simulink model "SecRwRtStFwdBkwdIsPosChk"  (R2024b)
settings: Solver=FixedStepDiscrete  StartTime=0.0  StopTime=10.0  FixedStep=0.01  RelTol=1e-3
undefined symbols (not defined in the file or in its folder): KeSMSuSecRwStFwdBkwdPosDelta_Val, KeSMSuSecRwStFwdBkwdPosTolr_Val
libraries: StIsPosChkLib x16, simulink x8
(part 2 of 2)

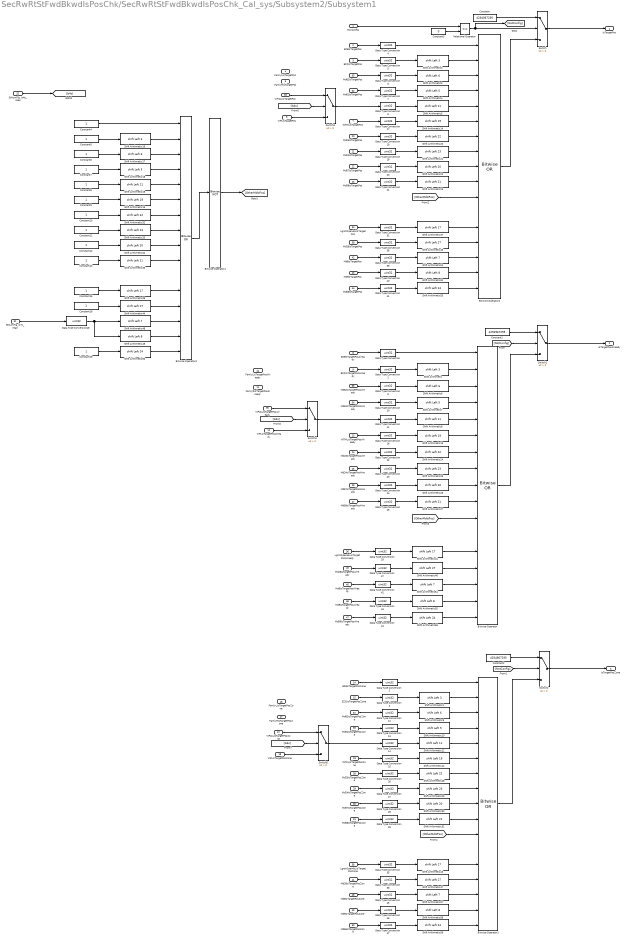
== system SecRwRtStFwdBkwdIsPosChk/SecRwRtStFwdBkwdIsPosChk_Cal_sys/Subsystem2/Subsystem1 ==
  MovConfig : Inport
  EZEIsTargetPos : Inport  Port=2
  EZQIsTargetPos : Inport  Port=3
  FamlyLIsTargetPos : Inport  Port=4
  FamlyRIsTargetPos : Inport  Port=5
  VIPLIsTargetPos : Inport  Port=6
  INTMLIsTargetPos : Inport  Port=7
  EZEIsTargetPosAlready : Inport  Port=8
  EZQIsTargetPosAlready : Inport  Port=9
  FamlyLIsTargetPosAlready : Inport  Port=10
  FamlyRIsTargetPosAlready : Inport  Port=11
  VIPLIsTargetPosAlready : Inport  Port=12
  INTMLIsTargetPosAlready : Inport  Port=13
  EZEIsTargetPosZone : Inport  Port=14
  EZQIsTargetPosZone : Inport  Port=15
  FamlyLIsTargetPosZone : Inport  Port=16
  FamlyRIsTargetPosZone : Inport  Port=17
  VIPLIsTargetPosZone : Inport  Port=18
  INTMLIsTargetPosZone : Inport  Port=19
  Md23IsTargetPos : Inport  Port=20
  Md24IsTargetPos : Inport  Port=21
  Md57IsTargetPos : Inport  Port=22
  Md58IsTargetPos : Inport  Port=23
  Md23IsTargetPosAlready : Inport  Port=24
  Md24IsTargetPosAlready : Inport  Port=25
  Md57IsTargetPosAlready : Inport  Port=26
  Md58IsTargetPosAlready : Inport  Port=27
  Md23IsTargetPosZone : Inport  Port=28
  Md24IsTargetPosZone : Inport  Port=29
  Md57IsTargetPosZone : Inport  Port=30
  Md58IsTargetPosZone : Inport  Port=31
  StNumFlg_Is4s_read : Inport  Port=32
  VIP4sLIsTargetPos : Inport  Port=33
  LgrstOpen4sLIsTargetPos : Inport  Port=34
  VIP4sLIsTargetPosAlready : Inport  Port=35
  LgrstOpen4sLIsTargetPosAlready : Inport  Port=36
  VIP4sLIsTargetPosZone : Inport  Port=37
  LgrstOpen4sLIsTargetPosZone : Inport  Port=38
  Md28IsTargetPos : Inport  Port=39
  Md28IsTargetPosAlready : Inport  Port=40
  Md28IsTargetPosZone : Inport  Port=41
  Md8IsTargetPos : Inport  Port=42
  Md9IsTargetPos : Inport  Port=43
  Md56IsTargetPos : Inport  Port=44
  Md8IsTargetPosAlready : Inport  Port=45
  Md9IsTargetPosAlready : Inport  Port=46
  Md56IsTargetPosAlready : Inport  Port=47
  Md8IsTargetPosZone : Inport  Port=48
  Md9IsTargetPosZone : Inport  Port=49
  Md56IsTargetPosZone : Inport  Port=50
  StNumFlg_Is7s_read : Inport  Port=51
  Md61IsTargetPos : Inport  Port=52
  Md62IsTargetPos : Inport  Port=53
  Md61IsTargetPosAlready : Inport  Port=54
  Md62IsTargetPosAlready : Inport  Port=55
  Md61IsTargetPosZone : Inport  Port=56
  Md62IsTargetPosZone : Inport  Port=57
  Bitwise Operator : simulink/Logic and Bit Operations/Bitwise Operator  logicop=OR  UseBitMask=off  NumInputPorts=17  BitMask=bin2dec('11011001')  BitMaskRealWorld=Stored Integer
  Bitwise Operator1 : simulink/Logic and Bit Operations/Bitwise Operator  logicop=OR  UseBitMask=off  NumInputPorts=17  BitMask=bin2dec('11011001')  BitMaskRealWorld=Stored Integer
  Bitwise Operator2 : simulink/Logic and Bit Operations/Bitwise Operator  logicop=OR  UseBitMask=off  NumInputPorts=17  BitMask=bin2dec('11011001')  BitMaskRealWorld=Stored Integer
  Bitwise Operator3 : simulink/Logic and Bit Operations/Bitwise Operator  logicop=OR  UseBitMask=off  NumInputPorts=16  BitMask=bin2dec('11011001')  BitMaskRealWorld=Stored Integer
  Bitwise Operator4 : simulink/Logic and Bit Operations/Bitwise Operator  logicop=NOT  UseBitMask=off  BitMask=bin2dec('11011001')  BitMaskRealWorld=Stored Integer
  Constant : Constant  Value=4294967295  OutDataTypeStr=uint32
  Constant1 : Constant  Value=4294967295  OutDataTypeStr=uint32
  Constant{4..13,15..16,19} (13 alike) : Constant  OutDataTypeStr=uint32
  Constant2 : Constant  Value=4294967295  OutDataTypeStr=uint32
  Constant3 : Constant  Value=0  OutDataTypeStr=uint8
  Data Type Conversion{,1..29,31,33,35..48} (46 alike) : DataTypeConversion  OutDataTypeStr=uint32  SaturateOnIntegerOverflow=off  RndMeth=Floor
  Relational Operator : RelationalOperator  Operator===  OutDataTypeStr=boolean  RndMeth=Simplest  InputSameDT=off
  Shift Arithmetic{,1..2,16} (4 alike) : ArithShift  BitShiftNumber=3  BitShiftDirection=Left
  Shift Arithmetic{4,7,10,18} (4 alike) : ArithShift  BitShiftNumber=5  BitShiftDirection=Left
  Shift Arithmetic{5,8,11,19} (4 alike) : ArithShift  BitShiftNumber=11  BitShiftDirection=Left
  Shift Arithmetic{12..15} (4 alike) : ArithShift  BitShiftNumber=19  BitShiftDirection=Left
  Shift Arithmetic{3,6,9,17} (4 alike) : ArithShift  BitShiftNumber=6  BitShiftDirection=Left
  Shift Arithmetic{20,24,28,32} (4 alike) : ArithShift  BitShiftNumber=22  BitShiftDirection=Left
  Shift Arithmetic{21,25,29,33} (4 alike) : ArithShift  BitShiftNumber=23  BitShiftDirection=Left
  Shift Arithmetic{22,26,30,34} (4 alike) : ArithShift  BitShiftNumber=20  BitShiftDirection=Left
  Shift Arithmetic{23,27,31,35} (4 alike) : ArithShift  BitShiftNumber=21  BitShiftDirection=Left
  Shift Arithmetic{37,39,41,43} (4 alike) : ArithShift  BitShiftNumber=17  BitShiftDirection=Left
  Shift Arithmetic{44..47} (4 alike) : ArithShift  BitShiftNumber=27  BitShiftDirection=Left
  Shift Arithmetic{48,51,54,57} (4 alike) : ArithShift  BitShiftNumber=7  BitShiftDirection=Left
  Shift Arithmetic{49,52,55,58} (4 alike) : ArithShift  BitShiftNumber=8  BitShiftDirection=Left
  Shift Arithmetic{50,53,56,59} (4 alike) : ArithShift  BitShiftNumber=24  BitShiftDirection=Left
  Switch{,1..5} (6 alike) : Switch  Criteria=u2 > Threshold  SaturateOnIntegerOverflow=off  InputSameDT=off
  IsTargetPos : Outport  VectorParamsAs1DForOutWhenUnconnected=off
      settings: EnsureOutportIsVirtual=on
  IsTargetPosAlready : Outport  Port=2  VectorParamsAs1DForOutWhenUnconnected=off
      settings: EnsureOutportIsVirtual=on
  IsTargetPosZone : Outport  Port=3  VectorParamsAs1DForOutWhenUnconnected=off
      settings: EnsureOutportIsVirtual=on
  wires:
  Constant3/1 -> Relational Operator/2
  Constant/1 -> Switch/1
  Relational Operator/1 -> [NotConfig], Switch/2
  MovConfig/1 -> Relational Operator/1
  Switch/1 -> IsTargetPos/1
  [NotConfig] -> Switch1/2
  Constant1/1 -> Switch1/1
  Switch1/1 -> IsTargetPosAlready/1
  Switch2/1 -> IsTargetPosZone/1
  Constant2/1 -> Switch2/1
  [NotConfig] -> Switch2/2
  Data Type Conversion1/1 -> Shift Arithmetic/1
  Data Type Conversion/1 -> Bitwise Operator/1
  Shift Arithmetic/1 -> Bitwise Operator/2
  Shift Arithmetic1/1 -> Bitwise Operator1/2
  Data Type Conversion2/1 -> Bitwise Operator1/1
  Data Type Conversion3/1 -> Shift Arithmetic1/1
  Bitwise Operator1/1 -> Switch2/3
  Bitwise Operator/1 -> Switch1/3
  Shift Arithmetic2/1 -> Bitwise Operator2/2
  Data Type Conversion4/1 -> Bitwise Operator2/1
  Data Type Conversion5/1 -> Shift Arithmetic2/1
  Bitwise Operator2/1 -> Switch/3
  EZEIsTargetPos/1 -> Data Type Conversion4/1
  EZQIsTargetPos/1 -> Data Type Conversion5/1
  EZQIsTargetPosZone/1 -> Data Type Conversion3/1
  EZEIsTargetPosZone/1 -> Data Type Conversion2/1
  EZQIsTargetPosAlready/1 -> Data Type Conversion1/1
  EZEIsTargetPosAlready/1 -> Data Type Conversion/1
  Shift Arithmetic3/1 -> Bitwise Operator2/3
  Shift Arithmetic4/1 -> Bitwise Operator2/4
  Shift Arithmetic5/1 -> Bitwise Operator2/5
  Data Type Conversion7/1 -> Shift Arithmetic4/1
  Data Type Conversion6/1 -> Shift Arithmetic3/1
  Data Type Conversion8/1 -> Shift Arithmetic5/1
  Data Type Conversion11/1 -> Shift Arithmetic8/1
  Data Type Conversion9/1 -> Shift Arithmetic6/1
  Data Type Conversion10/1 -> Shift Arithmetic7/1
  Shift Arithmetic8/1 -> Bitwise Operator/5
  Shift Arithmetic7/1 -> Bitwise Operator/4
  Shift Arithmetic6/1 -> Bitwise Operator/3
  Data Type Conversion14/1 -> Shift Arithmetic11/1
  Data Type Conversion13/1 -> Shift Arithmetic10/1
  Shift Arithmetic10/1 -> Bitwise Operator1/4
  Shift Arithmetic9/1 -> Bitwise Operator1/3
  Shift Arithmetic11/1 -> Bitwise Operator1/5
  Data Type Conversion12/1 -> Shift Arithmetic9/1
  Shift Arithmetic12/1 -> Bitwise Operator1/6
  Data Type Conversion15/1 -> Shift Arithmetic12/1
  INTMLIsTargetPosZone/1 -> Data Type Conversion15/1
  Shift Arithmetic13/1 -> Bitwise Operator/6
  Data Type Conversion16/1 -> Shift Arithmetic13/1
  INTMLIsTargetPosAlready/1 -> Data Type Conversion16/1
  Shift Arithmetic14/1 -> Bitwise Operator2/6
  Data Type Conversion17/1 -> Shift Arithmetic14/1
  INTMLIsTargetPos/1 -> Data Type Conversion17/1
  Shift Arithmetic15/1 -> Bitwise Operator3/6
  Shift Arithmetic18/1 -> Bitwise Operator3/4
  Shift Arithmetic17/1 -> Bitwise Operator3/3
  Bitwise Operator3/1 -> Bitwise Operator4/1
  Constant4/1 -> Bitwise Operator3/1
  Shift Arithmetic16/1 -> Bitwise Operator3/2
  Constant5/1 -> Shift Arithmetic16/1
  Constant6/1 -> Shift Arithmetic17/1
  Constant7/1 -> Shift Arithmetic18/1
  Constant8/1 -> Shift Arithmetic19/1
  Constant9/1 -> Shift Arithmetic15/1
  Bitwise Operator4/1 -> [OtherMdIsPos]
  [OtherMdIsPos] -> Bitwise Operator2/11
  Md23IsTargetPos/1 -> Data Type Conversion18/1
  Data Type Conversion18/1 -> Shift Arithmetic20/1
  Shift Arithmetic20/1 -> Bitwise Operator2/7
  Shift Arithmetic21/1 -> Bitwise Operator2/8
  Data Type Conversion19/1 -> Shift Arithmetic21/1
  Md24IsTargetPos/1 -> Data Type Conversion19/1
  Md57IsTargetPos/1 -> Data Type Conversion20/1
  Data Type Conversion20/1 -> Shift Arithmetic22/1
  Shift Arithmetic22/1 -> Bitwise Operator2/9
  Data Type Conversion21/1 -> Shift Arithmetic23/1
  Md58IsTargetPos/1 -> Data Type Conversion21/1
  Shift Arithmetic23/1 -> Bitwise Operator2/10
  [OtherMdIsPos] -> Bitwise Operator/11
  Md23IsTargetPosAlready/1 -> Data Type Conversion22/1
  Data Type Conversion22/1 -> Shift Arithmetic24/1
  Shift Arithmetic24/1 -> Bitwise Operator/7
  Shift Arithmetic25/1 -> Bitwise Operator/8
  Data Type Conversion23/1 -> Shift Arithmetic25/1
  Md24IsTargetPosAlready/1 -> Data Type Conversion23/1
  Md57IsTargetPosAlready/1 -> Data Type Conversion24/1
  Data Type Conversion24/1 -> Shift Arithmetic26/1
  Shift Arithmetic26/1 -> Bitwise Operator/9
  Shift Arithmetic27/1 -> Bitwise Operator/10
  Data Type Conversion25/1 -> Shift Arithmetic27/1
  Md58IsTargetPosAlready/1 -> Data Type Conversion25/1
  [OtherMdIsPos] -> Bitwise Operator1/11
  Md23IsTargetPosZone/1 -> Data Type Conversion26/1
  Data Type Conversion26/1 -> Shift Arithmetic28/1
  Shift Arithmetic28/1 -> Bitwise Operator1/7
  Shift Arithmetic29/1 -> Bitwise Operator1/8
  Data Type Conversion27/1 -> Shift Arithmetic29/1
  Md24IsTargetPosZone/1 -> Data Type Conversion27/1
  Md57IsTargetPosZone/1 -> Data Type Conversion28/1
  Data Type Conversion28/1 -> Shift Arithmetic30/1
  Shift Arithmetic30/1 -> Bitwise Operator1/9
  Shift Arithmetic31/1 -> Bitwise Operator1/10
  Data Type Conversion29/1 -> Shift Arithmetic31/1
  Md58IsTargetPosZone/1 -> Data Type Conversion29/1
  Constant10/1 -> Shift Arithmetic32/1
  Shift Arithmetic32/1 -> Bitwise Operator3/7
  Constant11/1 -> Shift Arithmetic33/1
  Shift Arithmetic33/1 -> Bitwise Operator3/8
  Shift Arithmetic34/1 -> Bitwise Operator3/9
  Constant12/1 -> Shift Arithmetic34/1
  Constant13/1 -> Shift Arithmetic35/1
  Shift Arithmetic35/1 -> Bitwise Operator3/10
  Shift Arithmetic19/1 -> Bitwise Operator3/5
  StNumFlg_Is4s_read/1 -> [Is4s]
  VIP4sLIsTargetPos/1 -> Switch3/1
  [Is4s] -> Switch3/2
  VIPLIsTargetPos/1 -> Switch3/3
  Switch3/1 -> Data Type Conversion8/1
  Data Type Conversion31/1 -> Shift Arithmetic37/1
  LgrstOpen4sLIsTargetPos/1 -> Data Type Conversion31/1
  Shift Arithmetic37/1 -> Bitwise Operator2/13
  Shift Arithmetic39/1 -> Bitwise Operator3/12
  Constant15/1 -> Shift Arithmetic39/1
  Switch4/1 -> Data Type Conversion11/1
  [Is4s] -> Switch4/2
  VIP4sLIsTargetPosAlready/1 -> Switch4/1
  VIPLIsTargetPosAlready/1 -> Switch4/3
  Shift Arithmetic41/1 -> Bitwise Operator/13
  LgrstOpen4sLIsTargetPosAlready/1 -> Data Type Conversion33/1
  Data Type Conversion33/1 -> Shift Arithmetic41/1
  Data Type Conversion35/1 -> Shift Arithmetic43/1
  LgrstOpen4sLIsTargetPosZone/1 -> Data Type Conversion35/1
  Shift Arithmetic43/1 -> Bitwise Operator1/13
  VIP4sLIsTargetPosZone/1 -> Switch5/1
  [Is4s] -> Switch5/2
  Switch5/1 -> Data Type Conversion14/1
  VIPLIsTargetPosZone/1 -> Switch5/3
  Constant16/1 -> Shift Arithmetic44/1
  Shift Arithmetic44/1 -> Bitwise Operator3/13
  Shift Arithmetic45/1 -> Bitwise Operator2/14
  Md28IsTargetPos/1 -> Data Type Conversion36/1
  Data Type Conversion36/1 -> Shift Arithmetic45/1
  Data Type Conversion37/1 -> Shift Arithmetic46/1
  Md28IsTargetPosAlready/1 -> Data Type Conversion37/1
  Shift Arithmetic46/1 -> Bitwise Operator/14
  Shift Arithmetic47/1 -> Bitwise Operator1/14
  Md28IsTargetPosZone/1 -> Data Type Conversion38/1
  Data Type Conversion38/1 -> Shift Arithmetic47/1
  Shift Arithmetic48/1 -> Bitwise Operator3/14
  Data Type Conversion48/1 -> Shift Arithmetic49/1, Shift Arithmetic48/1
  Shift Arithmetic49/1 -> Bitwise Operator3/15
  Shift Arithmetic50/1 -> Bitwise Operator3/16
  Constant19/1 -> Shift Arithmetic50/1
  Data Type Conversion39/1 -> Shift Arithmetic51/1
  Md8IsTargetPos/1 -> Data Type Conversion39/1
  Shift Arithmetic51/1 -> Bitwise Operator2/15
  Shift Arithmetic52/1 -> Bitwise Operator2/16
  Md9IsTargetPos/1 -> Data Type Conversion40/1
  Data Type Conversion40/1 -> Shift Arithmetic52/1
  Data Type Conversion41/1 -> Shift Arithmetic53/1
  Md56IsTargetPos/1 -> Data Type Conversion41/1
  Shift Arithmetic53/1 -> Bitwise Operator2/17
  Shift Arithmetic54/1 -> Bitwise Operator/15
  Md8IsTargetPosAlready/1 -> Data Type Conversion42/1
  Data Type Conversion42/1 -> Shift Arithmetic54/1
  Data Type Conversion43/1 -> Shift Arithmetic55/1
  Md9IsTargetPosAlready/1 -> Data Type Conversion43/1
  Shift Arithmetic55/1 -> Bitwise Operator/16
  Shift Arithmetic56/1 -> Bitwise Operator/17
  Md56IsTargetPosAlready/1 -> Data Type Conversion44/1
  Data Type Conversion44/1 -> Shift Arithmetic56/1
  Data Type Conversion45/1 -> Shift Arithmetic57/1
  Md8IsTargetPosZone/1 -> Data Type Conversion45/1
  Shift Arithmetic57/1 -> Bitwise Operator1/15
  Shift Arithmetic58/1 -> Bitwise Operator1/16
  Md9IsTargetPosZone/1 -> Data Type Conversion46/1
  Data Type Conversion46/1 -> Shift Arithmetic58/1
  Data Type Conversion47/1 -> Shift Arithmetic59/1
  Md56IsTargetPosZone/1 -> Data Type Conversion47/1
  Shift Arithmetic59/1 -> Bitwise Operator1/17
  StNumFlg_Is7s_read/1 -> Data Type Conversion48/1
  Md61IsTargetPos/1 -> Data Type Conversion7/1
  Md62IsTargetPos/1 -> Data Type Conversion6/1
  Md61IsTargetPosAlready/1 -> Data Type Conversion10/1
  Md62IsTargetPosAlready/1 -> Data Type Conversion9/1
  Md61IsTargetPosZone/1 -> Data Type Conversion13/1
  Md62IsTargetPosZone/1 -> Data Type Conversion12/1

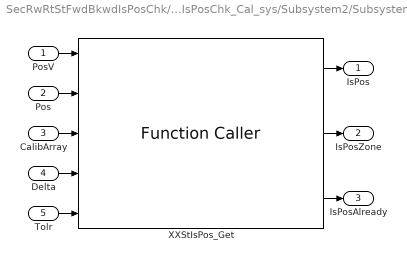
== system SecRwRtStFwdBkwdIsPosChk/SecRwRtStFwdBkwdIsPosChk_Cal_sys/Subsystem2/Subsystem10 ==
  PosV : Inport
  Pos : Inport  Port=2
  CalibArray : Inport  Port=3
  Delta : Inport  Port=4
  Tolr : Inport  Port=5
  XXStIsPos_Get : FunctionCaller  FunctionPrototype=[IsPos,IsPosZone,IsPosAlready] = XXStIsPos_Get(PosV,Pos,CalibArray,Delta,Tolr)  InputArgumentSpecifications=boolean(true), uint16(1), uint16([1;1;1]), uint16(1), uint16(1)  OutputArgumentSpecifications=boolean(true), boolean(true), boolean(true)
  IsPos : Outport  VectorParamsAs1DForOutWhenUnconnected=off
  IsPosZone : Outport  Port=2  VectorParamsAs1DForOutWhenUnconnected=off
  IsPosAlready : Outport  Port=3  VectorParamsAs1DForOutWhenUnconnected=off
  wires:
  Pos/1 -> XXStIsPos_Get/2
  PosV/1 -> XXStIsPos_Get/1
  XXStIsPos_Get/1 -> IsPos/1
  XXStIsPos_Get/2 -> IsPosZone/1
  CalibArray/1 -> XXStIsPos_Get/3
  XXStIsPos_Get/3 -> IsPosAlready/1
  Tolr/1 -> XXStIsPos_Get/5
  Delta/1 -> XXStIsPos_Get/4

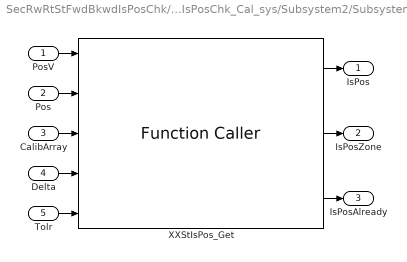
== system SecRwRtStFwdBkwdIsPosChk/SecRwRtStFwdBkwdIsPosChk_Cal_sys/Subsystem2/Subsystem11 ==
  PosV : Inport
  Pos : Inport  Port=2
  CalibArray : Inport  Port=3
  Delta : Inport  Port=4
  Tolr : Inport  Port=5
  XXStIsPos_Get : FunctionCaller  FunctionPrototype=[IsPos,IsPosZone,IsPosAlready] = XXStIsPos_Get(PosV,Pos,CalibArray,Delta,Tolr)  InputArgumentSpecifications=boolean(true), uint16(1), uint16([1;1;1]), uint16(1), uint16(1)  OutputArgumentSpecifications=boolean(true), boolean(true), boolean(true)
  IsPos : Outport  VectorParamsAs1DForOutWhenUnconnected=off
  IsPosZone : Outport  Port=2  VectorParamsAs1DForOutWhenUnconnected=off
  IsPosAlready : Outport  Port=3  VectorParamsAs1DForOutWhenUnconnected=off
  wires:
  Delta/1 -> XXStIsPos_Get/4
  Tolr/1 -> XXStIsPos_Get/5
  XXStIsPos_Get/3 -> IsPosAlready/1
  CalibArray/1 -> XXStIsPos_Get/3
  XXStIsPos_Get/2 -> IsPosZone/1
  XXStIsPos_Get/1 -> IsPos/1
  PosV/1 -> XXStIsPos_Get/1
  Pos/1 -> XXStIsPos_Get/2

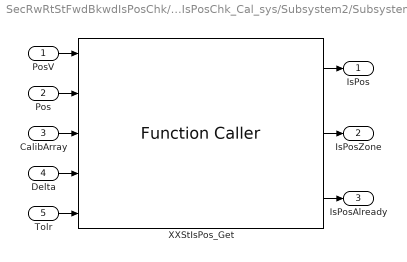
== system SecRwRtStFwdBkwdIsPosChk/SecRwRtStFwdBkwdIsPosChk_Cal_sys/Subsystem2/Subsystem12 ==
  PosV : Inport
  Pos : Inport  Port=2
  CalibArray : Inport  Port=3
  Delta : Inport  Port=4
  Tolr : Inport  Port=5
  XXStIsPos_Get : FunctionCaller  FunctionPrototype=[IsPos,IsPosZone,IsPosAlready] = XXStIsPos_Get(PosV,Pos,CalibArray,Delta,Tolr)  InputArgumentSpecifications=boolean(true), uint16(1), uint16([1;1;1]), uint16(1), uint16(1)  OutputArgumentSpecifications=boolean(true), boolean(true), boolean(true)
  IsPos : Outport  VectorParamsAs1DForOutWhenUnconnected=off
  IsPosZone : Outport  Port=2  VectorParamsAs1DForOutWhenUnconnected=off
  IsPosAlready : Outport  Port=3  VectorParamsAs1DForOutWhenUnconnected=off
  wires:
  Pos/1 -> XXStIsPos_Get/2
  PosV/1 -> XXStIsPos_Get/1
  XXStIsPos_Get/1 -> IsPos/1
  XXStIsPos_Get/2 -> IsPosZone/1
  CalibArray/1 -> XXStIsPos_Get/3
  XXStIsPos_Get/3 -> IsPosAlready/1
  Tolr/1 -> XXStIsPos_Get/5
  Delta/1 -> XXStIsPos_Get/4

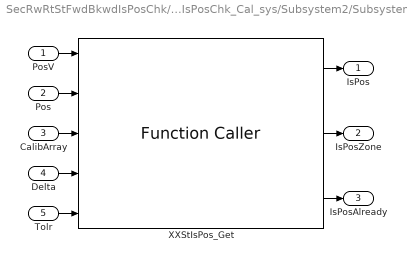
== system SecRwRtStFwdBkwdIsPosChk/SecRwRtStFwdBkwdIsPosChk_Cal_sys/Subsystem2/Subsystem13 ==
  PosV : Inport
  Pos : Inport  Port=2
  CalibArray : Inport  Port=3
  Delta : Inport  Port=4
  Tolr : Inport  Port=5
  XXStIsPos_Get : FunctionCaller  FunctionPrototype=[IsPos,IsPosZone,IsPosAlready] = XXStIsPos_Get(PosV,Pos,CalibArray,Delta,Tolr)  InputArgumentSpecifications=boolean(true), uint16(1), uint16([1;1;1]), uint16(1), uint16(1)  OutputArgumentSpecifications=boolean(true), boolean(true), boolean(true)
  IsPos : Outport  VectorParamsAs1DForOutWhenUnconnected=off
  IsPosZone : Outport  Port=2  VectorParamsAs1DForOutWhenUnconnected=off
  IsPosAlready : Outport  Port=3  VectorParamsAs1DForOutWhenUnconnected=off
  wires:
  Delta/1 -> XXStIsPos_Get/4
  Tolr/1 -> XXStIsPos_Get/5
  XXStIsPos_Get/3 -> IsPosAlready/1
  CalibArray/1 -> XXStIsPos_Get/3
  XXStIsPos_Get/2 -> IsPosZone/1
  XXStIsPos_Get/1 -> IsPos/1
  PosV/1 -> XXStIsPos_Get/1
  Pos/1 -> XXStIsPos_Get/2

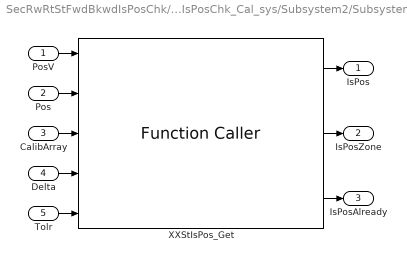
== system SecRwRtStFwdBkwdIsPosChk/SecRwRtStFwdBkwdIsPosChk_Cal_sys/Subsystem2/Subsystem14 ==
  PosV : Inport
  Pos : Inport  Port=2
  CalibArray : Inport  Port=3
  Delta : Inport  Port=4
  Tolr : Inport  Port=5
  XXStIsPos_Get : FunctionCaller  FunctionPrototype=[IsPos,IsPosZone,IsPosAlready] = XXStIsPos_Get(PosV,Pos,CalibArray,Delta,Tolr)  InputArgumentSpecifications=boolean(true), uint16(1), uint16([1;1;1]), uint16(1), uint16(1)  OutputArgumentSpecifications=boolean(true), boolean(true), boolean(true)
  IsPos : Outport  VectorParamsAs1DForOutWhenUnconnected=off
  IsPosZone : Outport  Port=2  VectorParamsAs1DForOutWhenUnconnected=off
  IsPosAlready : Outport  Port=3  VectorParamsAs1DForOutWhenUnconnected=off
  wires:
  Pos/1 -> XXStIsPos_Get/2
  PosV/1 -> XXStIsPos_Get/1
  XXStIsPos_Get/1 -> IsPos/1
  XXStIsPos_Get/2 -> IsPosZone/1
  CalibArray/1 -> XXStIsPos_Get/3
  XXStIsPos_Get/3 -> IsPosAlready/1
  Tolr/1 -> XXStIsPos_Get/5
  Delta/1 -> XXStIsPos_Get/4

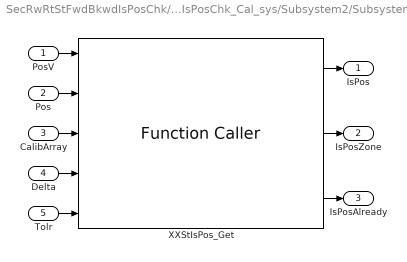
== system SecRwRtStFwdBkwdIsPosChk/SecRwRtStFwdBkwdIsPosChk_Cal_sys/Subsystem2/Subsystem15 ==
  PosV : Inport
  Pos : Inport  Port=2
  CalibArray : Inport  Port=3
  Delta : Inport  Port=4
  Tolr : Inport  Port=5
  XXStIsPos_Get : FunctionCaller  FunctionPrototype=[IsPos,IsPosZone,IsPosAlready] = XXStIsPos_Get(PosV,Pos,CalibArray,Delta,Tolr)  InputArgumentSpecifications=boolean(true), uint16(1), uint16([1;1;1]), uint16(1), uint16(1)  OutputArgumentSpecifications=boolean(true), boolean(true), boolean(true)
  IsPos : Outport  VectorParamsAs1DForOutWhenUnconnected=off
  IsPosZone : Outport  Port=2  VectorParamsAs1DForOutWhenUnconnected=off
  IsPosAlready : Outport  Port=3  VectorParamsAs1DForOutWhenUnconnected=off
  wires:
  Delta/1 -> XXStIsPos_Get/4
  Tolr/1 -> XXStIsPos_Get/5
  XXStIsPos_Get/3 -> IsPosAlready/1
  CalibArray/1 -> XXStIsPos_Get/3
  XXStIsPos_Get/2 -> IsPosZone/1
  XXStIsPos_Get/1 -> IsPos/1
  PosV/1 -> XXStIsPos_Get/1
  Pos/1 -> XXStIsPos_Get/2

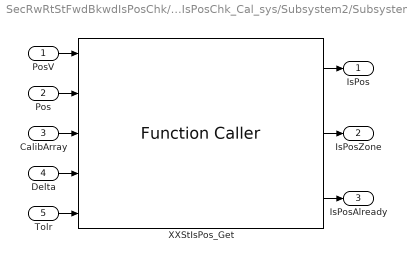
== system SecRwRtStFwdBkwdIsPosChk/SecRwRtStFwdBkwdIsPosChk_Cal_sys/Subsystem2/Subsystem16 ==
  PosV : Inport
  Pos : Inport  Port=2
  CalibArray : Inport  Port=3
  Delta : Inport  Port=4
  Tolr : Inport  Port=5
  XXStIsPos_Get : FunctionCaller  FunctionPrototype=[IsPos,IsPosZone,IsPosAlready] = XXStIsPos_Get(PosV,Pos,CalibArray,Delta,Tolr)  InputArgumentSpecifications=boolean(true), uint16(1), uint16([1;1;1]), uint16(1), uint16(1)  OutputArgumentSpecifications=boolean(true), boolean(true), boolean(true)
  IsPos : Outport  VectorParamsAs1DForOutWhenUnconnected=off
  IsPosZone : Outport  Port=2  VectorParamsAs1DForOutWhenUnconnected=off
  IsPosAlready : Outport  Port=3  VectorParamsAs1DForOutWhenUnconnected=off
  wires:
  Pos/1 -> XXStIsPos_Get/2
  PosV/1 -> XXStIsPos_Get/1
  XXStIsPos_Get/1 -> IsPos/1
  XXStIsPos_Get/2 -> IsPosZone/1
  CalibArray/1 -> XXStIsPos_Get/3
  XXStIsPos_Get/3 -> IsPosAlready/1
  Tolr/1 -> XXStIsPos_Get/5
  Delta/1 -> XXStIsPos_Get/4

== system SecRwRtStFwdBkwdIsPosChk/SecRwRtStFwdBkwdIsPosChk_Cal_sys/Subsystem2/Subsystem17 ==
  PosV : Inport
  Pos : Inport  Port=2
  CalibArray : Inport  Port=3
  Delta : Inport  Port=4
  Tolr : Inport  Port=5
  XXStIsPos_Get : FunctionCaller  FunctionPrototype=[IsPos,IsPosZone,IsPosAlready] = XXStIsPos_Get(PosV,Pos,CalibArray,Delta,Tolr)  InputArgumentSpecifications=boolean(true), uint16(1), uint16([1;1;1]), uint16(1), uint16(1)  OutputArgumentSpecifications=boolean(true), boolean(true), boolean(true)
  IsPos : Outport  VectorParamsAs1DForOutWhenUnconnected=off
  IsPosZone : Outport  Port=2  VectorParamsAs1DForOutWhenUnconnected=off
  IsPosAlready : Outport  Port=3  VectorParamsAs1DForOutWhenUnconnected=off
  wires:
  Delta/1 -> XXStIsPos_Get/4
  Tolr/1 -> XXStIsPos_Get/5
  XXStIsPos_Get/3 -> IsPosAlready/1
  CalibArray/1 -> XXStIsPos_Get/3
  XXStIsPos_Get/2 -> IsPosZone/1
  XXStIsPos_Get/1 -> IsPos/1
  PosV/1 -> XXStIsPos_Get/1
  Pos/1 -> XXStIsPos_Get/2

== system SecRwRtStFwdBkwdIsPosChk/SecRwRtStFwdBkwdIsPosChk_Cal_sys/Subsystem2/Subsystem18 ==
  PosV : Inport
  Pos : Inport  Port=2
  CalibArray : Inport  Port=3
  Delta : Inport  Port=4
  Tolr : Inport  Port=5
  XXStIsPos_Get : FunctionCaller  FunctionPrototype=[IsPos,IsPosZone,IsPosAlready] = XXStIsPos_Get(PosV,Pos,CalibArray,Delta,Tolr)  InputArgumentSpecifications=boolean(true), uint16(1), uint16([1;1;1]), uint16(1), uint16(1)  OutputArgumentSpecifications=boolean(true), boolean(true), boolean(true)
  IsPos : Outport  VectorParamsAs1DForOutWhenUnconnected=off
  IsPosZone : Outport  Port=2  VectorParamsAs1DForOutWhenUnconnected=off
  IsPosAlready : Outport  Port=3  VectorParamsAs1DForOutWhenUnconnected=off
  wires:
  Pos/1 -> XXStIsPos_Get/2
  PosV/1 -> XXStIsPos_Get/1
  XXStIsPos_Get/1 -> IsPos/1
  XXStIsPos_Get/2 -> IsPosZone/1
  CalibArray/1 -> XXStIsPos_Get/3
  XXStIsPos_Get/3 -> IsPosAlready/1
  Tolr/1 -> XXStIsPos_Get/5
  Delta/1 -> XXStIsPos_Get/4

== system SecRwRtStFwdBkwdIsPosChk/SecRwRtStFwdBkwdIsPosChk_Cal_sys/Subsystem2/Subsystem19 ==
  PosV : Inport
  Pos : Inport  Port=2
  CalibArray : Inport  Port=3
  Delta : Inport  Port=4
  Tolr : Inport  Port=5
  XXStIsPos_Get : FunctionCaller  FunctionPrototype=[IsPos,IsPosZone,IsPosAlready] = XXStIsPos_Get(PosV,Pos,CalibArray,Delta,Tolr)  InputArgumentSpecifications=boolean(true), uint16(1), uint16([1;1;1]), uint16(1), uint16(1)  OutputArgumentSpecifications=boolean(true), boolean(true), boolean(true)
  IsPos : Outport  VectorParamsAs1DForOutWhenUnconnected=off
  IsPosZone : Outport  Port=2  VectorParamsAs1DForOutWhenUnconnected=off
  IsPosAlready : Outport  Port=3  VectorParamsAs1DForOutWhenUnconnected=off
  wires:
  Delta/1 -> XXStIsPos_Get/4
  Tolr/1 -> XXStIsPos_Get/5
  XXStIsPos_Get/3 -> IsPosAlready/1
  CalibArray/1 -> XXStIsPos_Get/3
  XXStIsPos_Get/2 -> IsPosZone/1
  XXStIsPos_Get/1 -> IsPos/1
  PosV/1 -> XXStIsPos_Get/1
  Pos/1 -> XXStIsPos_Get/2

== system SecRwRtStFwdBkwdIsPosChk/SecRwRtStFwdBkwdIsPosChk_Cal_sys/Subsystem2/Subsystem2 ==
  PosV : Inport
  Pos : Inport  Port=2
  CalibArray : Inport  Port=3
  Delta : Inport  Port=4
  Tolr : Inport  Port=5
  XXStIsPos_Get : FunctionCaller  FunctionPrototype=[IsPos,IsPosZone,IsPosAlready] = XXStIsPos_Get(PosV,Pos,CalibArray,Delta,Tolr)  InputArgumentSpecifications=boolean(true), uint16(1), uint16([1;1;1]), uint16(1), uint16(1)  OutputArgumentSpecifications=boolean(true), boolean(true), boolean(true)
  IsPos : Outport  VectorParamsAs1DForOutWhenUnconnected=off
  IsPosZone : Outport  Port=2  VectorParamsAs1DForOutWhenUnconnected=off
  IsPosAlready : Outport  Port=3  VectorParamsAs1DForOutWhenUnconnected=off
  wires:
  Pos/1 -> XXStIsPos_Get/2
  PosV/1 -> XXStIsPos_Get/1
  XXStIsPos_Get/1 -> IsPos/1
  XXStIsPos_Get/2 -> IsPosZone/1
  CalibArray/1 -> XXStIsPos_Get/3
  XXStIsPos_Get/3 -> IsPosAlready/1
  Tolr/1 -> XXStIsPos_Get/5
  Delta/1 -> XXStIsPos_Get/4

== system SecRwRtStFwdBkwdIsPosChk/SecRwRtStFwdBkwdIsPosChk_Cal_sys/Subsystem2/Subsystem20 ==
  PosV : Inport
  Pos : Inport  Port=2
  CalibArray : Inport  Port=3
  Delta : Inport  Port=4
  Tolr : Inport  Port=5
  XXStIsPos_Get : FunctionCaller  FunctionPrototype=[IsPos,IsPosZone,IsPosAlready] = XXStIsPos_Get(PosV,Pos,CalibArray,Delta,Tolr)  InputArgumentSpecifications=boolean(true), uint16(1), uint16([1;1;1]), uint16(1), uint16(1)  OutputArgumentSpecifications=boolean(true), boolean(true), boolean(true)
  IsPos : Outport  VectorParamsAs1DForOutWhenUnconnected=off
  IsPosZone : Outport  Port=2  VectorParamsAs1DForOutWhenUnconnected=off
  IsPosAlready : Outport  Port=3  VectorParamsAs1DForOutWhenUnconnected=off
  wires:
  Pos/1 -> XXStIsPos_Get/2
  PosV/1 -> XXStIsPos_Get/1
  XXStIsPos_Get/1 -> IsPos/1
  XXStIsPos_Get/2 -> IsPosZone/1
  CalibArray/1 -> XXStIsPos_Get/3
  XXStIsPos_Get/3 -> IsPosAlready/1
  Tolr/1 -> XXStIsPos_Get/5
  Delta/1 -> XXStIsPos_Get/4

== system SecRwRtStFwdBkwdIsPosChk/SecRwRtStFwdBkwdIsPosChk_Cal_sys/Subsystem2/Subsystem21 ==
  PosV : Inport
  Pos : Inport  Port=2
  CalibArray : Inport  Port=3
  Delta : Inport  Port=4
  Tolr : Inport  Port=5
  XXStIsPos_Get : FunctionCaller  FunctionPrototype=[IsPos,IsPosZone,IsPosAlready] = XXStIsPos_Get(PosV,Pos,CalibArray,Delta,Tolr)  InputArgumentSpecifications=boolean(true), uint16(1), uint16([1;1;1]), uint16(1), uint16(1)  OutputArgumentSpecifications=boolean(true), boolean(true), boolean(true)
  IsPos : Outport  VectorParamsAs1DForOutWhenUnconnected=off
  IsPosZone : Outport  Port=2  VectorParamsAs1DForOutWhenUnconnected=off
  IsPosAlready : Outport  Port=3  VectorParamsAs1DForOutWhenUnconnected=off
  wires:
  Delta/1 -> XXStIsPos_Get/4
  Tolr/1 -> XXStIsPos_Get/5
  XXStIsPos_Get/3 -> IsPosAlready/1
  CalibArray/1 -> XXStIsPos_Get/3
  XXStIsPos_Get/2 -> IsPosZone/1
  XXStIsPos_Get/1 -> IsPos/1
  PosV/1 -> XXStIsPos_Get/1
  Pos/1 -> XXStIsPos_Get/2

== system SecRwRtStFwdBkwdIsPosChk/SecRwRtStFwdBkwdIsPosChk_Cal_sys/Subsystem2/Subsystem22 ==
  PosV : Inport
  Pos : Inport  Port=2
  CalibArray : Inport  Port=3
  Delta : Inport  Port=4
  Tolr : Inport  Port=5
  XXStIsPos_Get : FunctionCaller  FunctionPrototype=[IsPos,IsPosZone,IsPosAlready] = XXStIsPos_Get(PosV,Pos,CalibArray,Delta,Tolr)  InputArgumentSpecifications=boolean(true), uint16(1), uint16([1;1;1]), uint16(1), uint16(1)  OutputArgumentSpecifications=boolean(true), boolean(true), boolean(true)
  IsPos : Outport  VectorParamsAs1DForOutWhenUnconnected=off
  IsPosZone : Outport  Port=2  VectorParamsAs1DForOutWhenUnconnected=off
  IsPosAlready : Outport  Port=3  VectorParamsAs1DForOutWhenUnconnected=off
  wires:
  Pos/1 -> XXStIsPos_Get/2
  PosV/1 -> XXStIsPos_Get/1
  XXStIsPos_Get/1 -> IsPos/1
  XXStIsPos_Get/2 -> IsPosZone/1
  CalibArray/1 -> XXStIsPos_Get/3
  XXStIsPos_Get/3 -> IsPosAlready/1
  Tolr/1 -> XXStIsPos_Get/5
  Delta/1 -> XXStIsPos_Get/4

== system SecRwRtStFwdBkwdIsPosChk/SecRwRtStFwdBkwdIsPosChk_Cal_sys/Subsystem2/Subsystem3 ==
  PosV : Inport
  Pos : Inport  Port=2
  CalibArray : Inport  Port=3
  Delta : Inport  Port=4
  Tolr : Inport  Port=5
  XXStIsPos_Get : FunctionCaller  FunctionPrototype=[IsPos,IsPosZone,IsPosAlready] = XXStIsPos_Get(PosV,Pos,CalibArray,Delta,Tolr)  InputArgumentSpecifications=boolean(true), uint16(1), uint16([1;1;1]), uint16(1), uint16(1)  OutputArgumentSpecifications=boolean(true), boolean(true), boolean(true)
  IsPos : Outport  VectorParamsAs1DForOutWhenUnconnected=off
  IsPosZone : Outport  Port=2  VectorParamsAs1DForOutWhenUnconnected=off
  IsPosAlready : Outport  Port=3  VectorParamsAs1DForOutWhenUnconnected=off
  wires:
  Delta/1 -> XXStIsPos_Get/4
  Tolr/1 -> XXStIsPos_Get/5
  XXStIsPos_Get/3 -> IsPosAlready/1
  CalibArray/1 -> XXStIsPos_Get/3
  XXStIsPos_Get/2 -> IsPosZone/1
  XXStIsPos_Get/1 -> IsPos/1
  PosV/1 -> XXStIsPos_Get/1
  Pos/1 -> XXStIsPos_Get/2

== system SecRwRtStFwdBkwdIsPosChk/SecRwRtStFwdBkwdIsPosChk_Cal_sys/Subsystem2/Subsystem4 ==
  PosV : Inport
  Pos : Inport  Port=2
  CalibArray : Inport  Port=3
  Delta : Inport  Port=4
  Tolr : Inport  Port=5
  XXStIsPos_Get : FunctionCaller  FunctionPrototype=[IsPos,IsPosZone,IsPosAlready] = XXStIsPos_Get(PosV,Pos,CalibArray,Delta,Tolr)  InputArgumentSpecifications=boolean(true), uint16(1), uint16([1;1;1]), uint16(1), uint16(1)  OutputArgumentSpecifications=boolean(true), boolean(true), boolean(true)
  IsPos : Outport  VectorParamsAs1DForOutWhenUnconnected=off
  IsPosZone : Outport  Port=2  VectorParamsAs1DForOutWhenUnconnected=off
  IsPosAlready : Outport  Port=3  VectorParamsAs1DForOutWhenUnconnected=off
  wires:
  Pos/1 -> XXStIsPos_Get/2
  PosV/1 -> XXStIsPos_Get/1
  XXStIsPos_Get/1 -> IsPos/1
  XXStIsPos_Get/2 -> IsPosZone/1
  CalibArray/1 -> XXStIsPos_Get/3
  XXStIsPos_Get/3 -> IsPosAlready/1
  Tolr/1 -> XXStIsPos_Get/5
  Delta/1 -> XXStIsPos_Get/4

== system SecRwRtStFwdBkwdIsPosChk/SecRwRtStFwdBkwdIsPosChk_Cal_sys/Subsystem2/Subsystem5 ==
  PosV : Inport
  Pos : Inport  Port=2
  CalibArray : Inport  Port=3
  Delta : Inport  Port=4
  Tolr : Inport  Port=5
  XXStIsPos_Get : FunctionCaller  FunctionPrototype=[IsPos,IsPosZone,IsPosAlready] = XXStIsPos_Get(PosV,Pos,CalibArray,Delta,Tolr)  InputArgumentSpecifications=boolean(true), uint16(1), uint16([1;1;1]), uint16(1), uint16(1)  OutputArgumentSpecifications=boolean(true), boolean(true), boolean(true)
  IsPos : Outport  VectorParamsAs1DForOutWhenUnconnected=off
  IsPosZone : Outport  Port=2  VectorParamsAs1DForOutWhenUnconnected=off
  IsPosAlready : Outport  Port=3  VectorParamsAs1DForOutWhenUnconnected=off
  wires:
  Delta/1 -> XXStIsPos_Get/4
  Tolr/1 -> XXStIsPos_Get/5
  XXStIsPos_Get/3 -> IsPosAlready/1
  CalibArray/1 -> XXStIsPos_Get/3
  XXStIsPos_Get/2 -> IsPosZone/1
  XXStIsPos_Get/1 -> IsPos/1
  PosV/1 -> XXStIsPos_Get/1
  Pos/1 -> XXStIsPos_Get/2

== system SecRwRtStFwdBkwdIsPosChk/SecRwRtStFwdBkwdIsPosChk_Cal_sys/Subsystem2/Subsystem6 ==
  PosV : Inport
  Pos : Inport  Port=2
  CalibArray : Inport  Port=3
  Delta : Inport  Port=4
  Tolr : Inport  Port=5
  XXStIsPos_Get : FunctionCaller  FunctionPrototype=[IsPos,IsPosZone,IsPosAlready] = XXStIsPos_Get(PosV,Pos,CalibArray,Delta,Tolr)  InputArgumentSpecifications=boolean(true), uint16(1), uint16([1;1;1]), uint16(1), uint16(1)  OutputArgumentSpecifications=boolean(true), boolean(true), boolean(true)
  IsPos : Outport  VectorParamsAs1DForOutWhenUnconnected=off
  IsPosZone : Outport  Port=2  VectorParamsAs1DForOutWhenUnconnected=off
  IsPosAlready : Outport  Port=3  VectorParamsAs1DForOutWhenUnconnected=off
  wires:
  Pos/1 -> XXStIsPos_Get/2
  PosV/1 -> XXStIsPos_Get/1
  XXStIsPos_Get/1 -> IsPos/1
  XXStIsPos_Get/2 -> IsPosZone/1
  CalibArray/1 -> XXStIsPos_Get/3
  XXStIsPos_Get/3 -> IsPosAlready/1
  Tolr/1 -> XXStIsPos_Get/5
  Delta/1 -> XXStIsPos_Get/4

== system SecRwRtStFwdBkwdIsPosChk/SecRwRtStFwdBkwdIsPosChk_Cal_sys/Subsystem2/Subsystem7 ==
  PosV : Inport
  Pos : Inport  Port=2
  CalibArray : Inport  Port=3
  Delta : Inport  Port=4
  Tolr : Inport  Port=5
  XXStIsPos_Get : FunctionCaller  FunctionPrototype=[IsPos,IsPosZone,IsPosAlready] = XXStIsPos_Get(PosV,Pos,CalibArray,Delta,Tolr)  InputArgumentSpecifications=boolean(true), uint16(1), uint16([1;1;1]), uint16(1), uint16(1)  OutputArgumentSpecifications=boolean(true), boolean(true), boolean(true)
  IsPos : Outport  VectorParamsAs1DForOutWhenUnconnected=off
  IsPosZone : Outport  Port=2  VectorParamsAs1DForOutWhenUnconnected=off
  IsPosAlready : Outport  Port=3  VectorParamsAs1DForOutWhenUnconnected=off
  wires:
  Delta/1 -> XXStIsPos_Get/4
  Tolr/1 -> XXStIsPos_Get/5
  XXStIsPos_Get/3 -> IsPosAlready/1
  CalibArray/1 -> XXStIsPos_Get/3
  XXStIsPos_Get/2 -> IsPosZone/1
  XXStIsPos_Get/1 -> IsPos/1
  PosV/1 -> XXStIsPos_Get/1
  Pos/1 -> XXStIsPos_Get/2

== system SecRwRtStFwdBkwdIsPosChk/SecRwRtStFwdBkwdIsPosChk_Cal_sys/Subsystem2/Subsystem8 ==
  PosV : Inport
  Pos : Inport  Port=2
  CalibArray : Inport  Port=3
  Delta : Inport  Port=4
  Tolr : Inport  Port=5
  XXStIsPos_Get : FunctionCaller  FunctionPrototype=[IsPos,IsPosZone,IsPosAlready] = XXStIsPos_Get(PosV,Pos,CalibArray,Delta,Tolr)  InputArgumentSpecifications=boolean(true), uint16(1), uint16([1;1;1]), uint16(1), uint16(1)  OutputArgumentSpecifications=boolean(true), boolean(true), boolean(true)
  IsPos : Outport  VectorParamsAs1DForOutWhenUnconnected=off
  IsPosZone : Outport  Port=2  VectorParamsAs1DForOutWhenUnconnected=off
  IsPosAlready : Outport  Port=3  VectorParamsAs1DForOutWhenUnconnected=off
  wires:
  Pos/1 -> XXStIsPos_Get/2
  PosV/1 -> XXStIsPos_Get/1
  XXStIsPos_Get/1 -> IsPos/1
  XXStIsPos_Get/2 -> IsPosZone/1
  CalibArray/1 -> XXStIsPos_Get/3
  XXStIsPos_Get/3 -> IsPosAlready/1
  Tolr/1 -> XXStIsPos_Get/5
  Delta/1 -> XXStIsPos_Get/4

== system SecRwRtStFwdBkwdIsPosChk/SecRwRtStFwdBkwdIsPosChk_Cal_sys/Subsystem2/Subsystem9 ==
  PosV : Inport
  Pos : Inport  Port=2
  CalibArray : Inport  Port=3
  Delta : Inport  Port=4
  Tolr : Inport  Port=5
  XXStIsPos_Get : FunctionCaller  FunctionPrototype=[IsPos,IsPosZone,IsPosAlready] = XXStIsPos_Get(PosV,Pos,CalibArray,Delta,Tolr)  InputArgumentSpecifications=boolean(true), uint16(1), uint16([1;1;1]), uint16(1), uint16(1)  OutputArgumentSpecifications=boolean(true), boolean(true), boolean(true)
  IsPos : Outport  VectorParamsAs1DForOutWhenUnconnected=off
  IsPosZone : Outport  Port=2  VectorParamsAs1DForOutWhenUnconnected=off
  IsPosAlready : Outport  Port=3  VectorParamsAs1DForOutWhenUnconnected=off
  wires:
  Delta/1 -> XXStIsPos_Get/4
  Tolr/1 -> XXStIsPos_Get/5
  XXStIsPos_Get/3 -> IsPosAlready/1
  CalibArray/1 -> XXStIsPos_Get/3
  XXStIsPos_Get/2 -> IsPosZone/1
  XXStIsPos_Get/1 -> IsPos/1
  PosV/1 -> XXStIsPos_Get/1
  Pos/1 -> XXStIsPos_Get/2
